simulink model "CrashAlgo_TestEnvironment_DU_v2"  (R2019a)
settings: Solver=FixedStepDiscrete  StartTime=0.0  StopTime=t(end)  FixedStep=0.001  RelTol=1e-3
undefined symbols (not defined in the file or in its folder): BDU250_CRCL_DWork_DU_speed_kmh, BDU250_CRCL_DWork_HD_CollisionHitFire, BDU250_CRCL_DWork_HD_GroundHitFire, BDU250_CRCL_DWork_HD_strongCollisionFire, BDU250_CRCL_DWork_pitchKalman_deg, BDU250_CRCL_DWork_RD_fire, BDU250_CRCL_DWork_rollKalman_deg, BDU250_CRCL_DWork_SD_StandFire, BDU250_CRCL_DWork_TO_fire, BDU250_CRCL_scenario, BDU250_ROID_accBfXMg, BDU250_ROID_accBfYMg, BDU250_ROID_accBfZMg, BDU250_ROID_gyrBfXMdegs, BDU250_ROID_gyrBfYMdegs, BDU250_ROID_gyrBfZMdegs, CAN1_DU_BikeSpeed_PresentBikeSpeedHmi, CAN1_DU_DriverInfo_DriverCadence
settings Model: DataTypeOverride=Off  DataTypeOverrideAppliesTo=Floating-point  MinMaxOverflowLogging=ForceOff  Creator=stj1si  LastModifiedBy=snj7rt
settings DataIOCC: SaveFormat=Array  SaveOutput=off  SignalLogging=off  SaveTime=off  ReturnWorkspaceOutputs=off
settings OptimizationCC: DefaultParameterBehavior=Inlined  DefaultUnderspecifiedDataType=single  InlineInvariantSignals=on  EnhancedBackFolding=on  CachingGlobalReferences=on  ExpressionDepthLimit=2147483647  NoFixptDivByZeroProtection=on  EfficientFloat2IntCast=on  LifeSpan=1  SimCompilerOptimization=on
settings DebuggingCC: SolverPrmCheckMsg=warning  AllowSymbolicDim=off  StateNameClashWarn=warning  SFUnexpectedBacktrackingDiag=warning  SFNoUnconditionalDefaultTransitionDiag=warning  SFExecutionAtInitializationDiag=none  ArithmeticOperatorsInVariantConditions=warning
settings HardwareCC: ProdBitPerPointer=32  ProdBitPerSizeT=32  ProdBitPerPtrDiffT=32  ProdLargestAtomicInteger=Long  ProdLargestAtomicFloat=Double  ProdEndianess=BigEndian  ProdWordSize=32  ProdHWDeviceType=Freescale->32-bit PowerPC
settings ModelReferenceCC: ModelReferenceNumInstancesAllowed=Single  PropagateSignalLabelsOutOfModel=off
settings SFSimCC: SimUseLocalCustomCode=off  MATLABDynamicMemAlloc=off
settings RTWCC: SystemTargetFile=ert.tlc  GenCodeOnly=on  TemplateMakefile=ert_default_tmf  GenerateReport=on  RTWUseLocalCustomCode=off  IncludeHyperlinkInReport=on  LaunchReport=on  GenerateTraceInfo=on  GenerateTraceReport=on  GenerateTraceReportSl=on  GenerateTraceReportSf=on  GenerateTraceReportEml=on
settings CodeAppCC: IgnoreCustomStorageClasses=off  CustomSymbolStrType=$N$R$M  CustomSymbolStrBlkIO=CADE_rtb_$N$M  StateflowObjectComments=on  InternalIdentifier=Classic
settings ERTTargetCC: TargetLangStandard=C99 (ISO)  MultiwordLength=2048  GenerateSampleERTMain=on  IncludeMdlTerminateFcn=off  CombineSignalStateStructs=on  SuppressErrorStatus=on  SupportNonFinite=off  SupportComplex=off  CastingMode=Standards  InlinedParameterPlacement=NonHierarchical  ERTSrcFileBannerTemplate=ert_code_template_ebike.cgt  ERTCustomFileTemplate=example_file_process.tlc  ERTFilePackagingFormat=Compact  PreserveExternInFcnDecls=off  SuppressUnreachableDefaultCases=off  EnableSignedLeftShifts=off  EnableSignedRightShifts=off  IndentStyle=Allman  EnableUserReplacementTypes=on
settings ConfigComp: CovMetricSettings=dw  CovHTMLOptions=-sRT=1 -sVT=0 -aTS=1 -bRG=1 -bTC=1 -hTR=0 -nFC=0 -nFD=1 -scm=1 -bcm=1 -xEv=0 -xEM=0  CovHtmlReporting=on  CovSaveCumulativeToWorkspaceVar=on  CovSaveSingleToWorkspaceVar=on  CovSFcnEnable=off

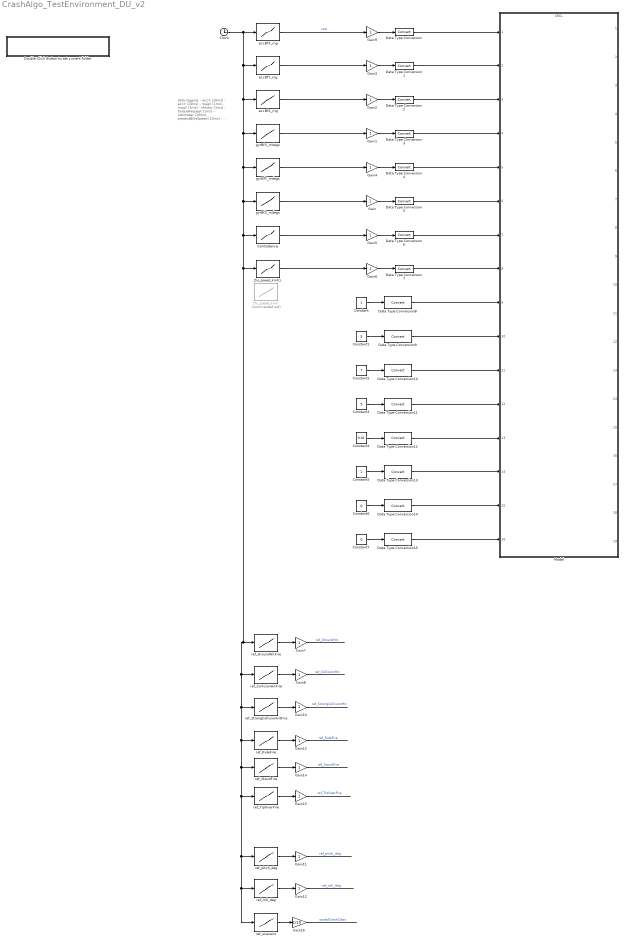
== system CrashAlgo_TestEnvironment_DU_v2 ==
  note: data logging:
      | - accX (10ms)
      | - accY (10ms)
      | - magX (1ms)
      | - magY (1ms)
      | - nMotor (1ms)
      | - torqueRequest (1ms)
      | - odometer (10ms)
      | - presentBikeSpeed (10ms)
      | - installationAngle (500ms)
  CanCadence : Lookup_n-D  NumberOfTableDimensions=1  BreakpointsForDimension1=t  Table=CAN1_DU_DriverInfo_DriverCadence  InterpMethod=Flat  InternalRulePriority=Speed  RndMeth=Simplest  InputSameDT=on
  Clock : Clock
  Constant : Constant
  Constant1 : Constant  Value=5
  Constant2 : Constant  Value=7
  Constant3 : Constant  Value=5
  Constant4 : Constant  Value=0.01
  Constant5 : Constant
  Constant6 : Constant  Value=0
  Constant7 : Constant  Value=0
  Data Type Conversion{,1..15} (16 alike) : DataTypeConversion
  Double-Click Button to set current folder : Subsystem
      settings: OpenFcn=cd(fileparts(get_param(gcs,'filename')));
      mask Display: disp('\bf\fontsize{16}Double-Click to set current folder      ','texmode','on')
  Du_speed_kmh : Lookup_n-D  Commented=on  NumberOfTableDimensions=1  BreakpointsForDimension1=t  Table=BDU250_CRCL_DWork_DU_speed_kmh  InterpMethod=Flat  InternalRulePriority=Speed  RndMeth=Simplest  InputSameDT=on
  Du_speed_kmh1 : Lookup_n-D  NumberOfTableDimensions=1  BreakpointsForDimension1=t  Table=CAN1_DU_BikeSpeed_PresentBikeSpeedHmi  InterpMethod=Flat  InternalRulePriority=Speed  RndMeth=Simplest  InputSameDT=on
  Gain{,1..15} (16 alike) : Gain
      settings: AttributesFormatString=%<Gain>
  Gain16 : Gain  Gain=1/10
      settings: AttributesFormatString=%<Gain>
  Model : ModelReference  ModelNameDialog=CRCL.slx  SimulationMode=Normal  ModelReferenceVersion=1.1836
  accBfX_mg : Lookup_n-D  NumberOfTableDimensions=1  BreakpointsForDimension1=t  Table=BDU250_ROID_accBfXMg  InterpMethod=Flat  InternalRulePriority=Speed  RndMeth=Simplest  InputSameDT=on
  accBfY_mg : Lookup_n-D  NumberOfTableDimensions=1  BreakpointsForDimension1=t  Table=BDU250_ROID_accBfYMg  InterpMethod=Flat  InternalRulePriority=Speed  RndMeth=Simplest  InputSameDT=on
  accBfZ_mg : Lookup_n-D  NumberOfTableDimensions=1  BreakpointsForDimension1=t  Table=BDU250_ROID_accBfZMg  InterpMethod=Flat  InternalRulePriority=Speed  RndMeth=Simplest  InputSameDT=on
  gyrBfX_mdegs : Lookup_n-D  NumberOfTableDimensions=1  BreakpointsForDimension1=t  Table=BDU250_ROID_gyrBfXMdegs  InterpMethod=Flat  InternalRulePriority=Speed  RndMeth=Simplest  InputSameDT=on
  gyrBfY_mdegs : Lookup_n-D  NumberOfTableDimensions=1  BreakpointsForDimension1=t  Table=BDU250_ROID_gyrBfYMdegs  InterpMethod=Flat  InternalRulePriority=Speed  RndMeth=Simplest  InputSameDT=on
  gyrBfZ_mdegs : Lookup_n-D  NumberOfTableDimensions=1  BreakpointsForDimension1=t  Table=BDU250_ROID_gyrBfZMdegs  InterpMethod=Flat  InternalRulePriority=Speed  RndMeth=Simplest  InputSameDT=on
  ref_CollisionHitFire : Lookup_n-D  NumberOfTableDimensions=1  BreakpointsForDimension1=t  Table=BDU250_CRCL_DWork_HD_CollisionHitFire  InterpMethod=Flat  InternalRulePriority=Speed  RndMeth=Simplest  InputSameDT=on
  ref_GroundHitFire : Lookup_n-D  NumberOfTableDimensions=1  BreakpointsForDimension1=t  Table=BDU250_CRCL_DWork_HD_GroundHitFire  InterpMethod=Flat  InternalRulePriority=Speed  RndMeth=Simplest  InputSameDT=on
  ref_RideFire : Lookup_n-D  NumberOfTableDimensions=1  BreakpointsForDimension1=t  Table=BDU250_CRCL_DWork_RD_fire  InterpMethod=Flat  InternalRulePriority=Speed  RndMeth=Simplest  InputSameDT=on
  ref_StandFire : Lookup_n-D  NumberOfTableDimensions=1  BreakpointsForDimension1=t  Table=BDU250_CRCL_DWork_SD_StandFire  InterpMethod=Flat  InternalRulePriority=Speed  RndMeth=Simplest  InputSameDT=on
  ref_StrongCollisionHitFire : Lookup_n-D  NumberOfTableDimensions=1  BreakpointsForDimension1=t  Table=BDU250_CRCL_DWork_HD_strongCollisionFire  InterpMethod=Flat  InternalRulePriority=Speed  RndMeth=Simplest  InputSameDT=on
  ref_TipOverFire : Lookup_n-D  NumberOfTableDimensions=1  BreakpointsForDimension1=t  Table=BDU250_CRCL_DWork_TO_fire  InterpMethod=Flat  InternalRulePriority=Speed  RndMeth=Simplest  InputSameDT=on
  ref_pitch_deg : Lookup_n-D  NumberOfTableDimensions=1  BreakpointsForDimension1=t  Table=BDU250_CRCL_DWork_pitchKalman_deg  InterpMethod=Flat  InternalRulePriority=Speed  RndMeth=Simplest  InputSameDT=on
  ref_roll_deg : Lookup_n-D  NumberOfTableDimensions=1  BreakpointsForDimension1=t  Table=BDU250_CRCL_DWork_rollKalman_deg  InterpMethod=Flat  InternalRulePriority=Speed  RndMeth=Simplest  InputSameDT=on
  ref_scenario : Lookup_n-D  NumberOfTableDimensions=1  BreakpointsForDimension1=t  Table=BDU250_CRCL_scenario  InterpMethod=Flat  InternalRulePriority=Speed  RndMeth=Simplest  InputSameDT=on
  wires:
  accBfX_mg/1 -> Gain9/1  "raw"
  accBfY_mg/1 -> Gain3/1
  gyrBfY_mdegs/1 -> Gain4/1
  gyrBfZ_mdegs/1 -> Gain/1
  Gain3/1 -> Data Type Conversion1/1
  Gain2/1 -> Data Type Conversion2/1
  gyrBfX_mdegs/1 -> Gain1/1
  Gain9/1 -> Data Type Conversion/1
  Gain4/1 -> Data Type Conversion4/1
  Gain/1 -> Data Type Conversion5/1
  CanCadence/1 -> Gain5/1
  Gain1/1 -> Data Type Conversion3/1
  Gain5/1 -> Data Type Conversion6/1
  Gain6/1 -> Data Type Conversion7/1
  Gain7/1 -> ?  "ref_GroundHit"
  Data Type Conversion/1 -> Model/1
  Data Type Conversion1/1 -> Model/2
  Data Type Conversion2/1 -> Model/3
  Data Type Conversion3/1 -> Model/4
  Data Type Conversion4/1 -> Model/5
  Data Type Conversion5/1 -> Model/6
  Data Type Conversion6/1 -> Model/7
  Du_speed_kmh1/1 -> Gain6/1
  Data Type Conversion7/1 -> Model/8
  ref_GroundHitFire/1 -> Gain7/1
  ref_CollisionHitFire/1 -> Gain8/1
  Gain8/1 -> ?  "ref_CollisionHit"
  Gain10/1 -> ?  "ref_StrongCollisionHit"
  ref_StrongCollisionHitFire/1 -> Gain10/1
  ref_pitch_deg/1 -> Gain11/1
  Gain11/1 -> ?  "ref_pitch_deg"
  Clock/1 -> accBfX_mg/1, accBfY_mg/1, accBfZ_mg/1, gyrBfX_mdegs/1, gyrBfY_mdegs/1, gyrBfZ_mdegs/1, CanCadence/1, Du_speed_kmh1/1, ref_GroundHitFire/1, ref_StrongCollisionHitFire/1, ref_RideFire/1, ref_StandFire/1, ref_TipOverFire/1, ref_pitch_deg/1, ref_roll_deg/1, ref_scenario/1, ref_CollisionHitFire/1
  Gain12/1 -> ?  "ref_roll_deg"
  ref_roll_deg/1 -> Gain12/1
  ref_RideFire/1 -> Gain13/1
  Gain13/1 -> ?  "ref_RideFire"
  Gain14/1 -> ?  "ref_StandFire"
  ref_StandFire/1 -> Gain14/1
  ref_TipOverFire/1 -> Gain15/1
  Gain15/1 -> ?  "ref_TipOverFire"
  Gain16/1 -> ?  "savedCrashClass"
  ref_scenario/1 -> Gain16/1
  Data Type Conversion8/1 -> Model/9
  Constant/1 -> Data Type Conversion8/1
  Constant1/1 -> Data Type Conversion9/1
  Data Type Conversion9/1 -> Model/10
  Constant2/1 -> Data Type Conversion10/1
  Data Type Conversion10/1 -> Model/11
  Constant3/1 -> Data Type Conversion11/1
  Data Type Conversion11/1 -> Model/12
  Constant4/1 -> Data Type Conversion12/1
  Data Type Conversion12/1 -> Model/13
  accBfZ_mg/1 -> Gain2/1
  Data Type Conversion13/1 -> Model/14
  Constant5/1 -> Data Type Conversion13/1
  Constant6/1 -> Data Type Conversion14/1
  Data Type Conversion14/1 -> Model/15
  Constant7/1 -> Data Type Conversion15/1
  Data Type Conversion15/1 -> Model/16

== system CrashAlgo_TestEnvironment_DU_v2/Double-Click Button to set current folder ==
